simulink model "KalmanFilterSimulation"  (Simulink 6.4)
settings: Solver=ode45  StartTime=0.0  StopTime=100  RelTol=1e-3
values from neighbouring files (symbols this model uses):
  A = [-0.01357 -32.2 -46.3 0 ... (first row only)    [ZeroSetpointLQR.m]    (also in nonZeroSetpointLQR.m; part1b.m)
  B = [-0.433;0.1394;-0.1394;-0.1577]    [ZeroSetpointLQR.m]    (also in nonZeroSetpointLQR.m; part1b.m)
  C = eye(n)    [ZeroSetpointLQR.m]    (also in nonZeroSetpointLQR.m; part1b.m)
  n = 4    [ZeroSetpointLQR.m]    (also in nonZeroSetpointLQR.m; part1b.m)
  r = 10    [nonZeroSetpointLQR.m]    (also in part1b.m)
  x0 = [1;1;1;1]    [ZeroSetpointLQR.m]    (also in nonZeroSetpointLQR.m; part1b.m)
undefined symbols (not defined in the file or in its folder): F, G, K, m1, m2, W2
libraries: simulink x3
settings Model: LastModifiedBy=Admin

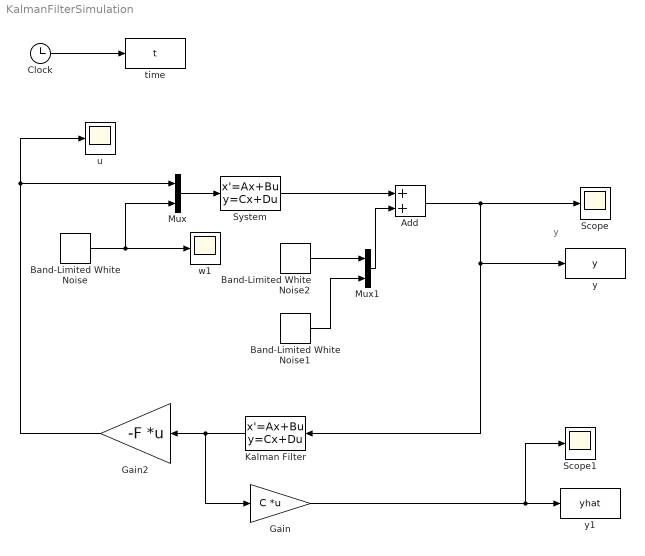
== system KalmanFilterSimulation ==
  note: y
  Add : Sum  OutScaling=2^-10
  Band-Limited White Noise : simulink/Sources/Band-Limited White Noise  SystemSampleTime=-1  Cov=W1  Ts=0.001  seed=[23341]  VectorParams1D=off
  Band-Limited White Noise1 : simulink/Sources/Band-Limited White Noise  SystemSampleTime=-1  Cov=W2(2,2)  Ts=0.001  seed=[23341]  VectorParams1D=off
  Band-Limited White Noise2 : simulink/Sources/Band-Limited White Noise  SystemSampleTime=-1  Cov=W2(1,1)  Ts=0.001  seed=[23341]  VectorParams1D=off
  Clock : Clock
      settings: Decimation=10
  Gain : Gain  Gain=C  Multiplication=Matrix(K*u)
  Gain2 : Gain  Orientation=left  Gain=-F  Multiplication=Matrix(K*u)
  Kalman Filter : StateSpace  Orientation=left  A=A-K*C  B=K  C=eye(n)  D=zeros(n,2)  X0=x0
  Mux : Mux  Inputs=2
  Mux1 : Mux  Inputs=2
  Scope : Scope
  Scope1 : Scope
      settings: YMin=-375  YMax=25
  System : StateSpace  A=A  B=[B G]  C=C  D=zeros(r,m1+m2)  X0=x0
  time : ToWorkspace  VariableName=t  SampleTime=-1  SaveFormat=Array
  u : Scope
      settings: SaveName=ScopeData10
  w1 : Scope
      settings: YMin=-7  YMax=7  SaveName=ScopeData9
  y : ToWorkspace  VariableName=y  SampleTime=-1  SaveFormat=Array
  y1 : ToWorkspace  VariableName=yhat  SampleTime=-1  SaveFormat=Array
  wires:
  Band-Limited White Noise/1 -> Mux/2, w1/1
  Mux/1 -> System/1
  Clock/1 -> time/1
  Add/1 -> Scope/1, y/1, Kalman Filter/1
  System/1 -> Add/1
  Kalman Filter/1 -> Gain2/1, Gain/1
  Gain2/1 -> Mux/1, u/1
  Band-Limited White Noise2/1 -> Mux1/1
  Band-Limited White Noise1/1 -> Mux1/2
  Mux1/1 -> Add/2
  Gain/1 -> y1/1, Scope1/1
